simulink model "tracker_resize"  (Simulink 6.4)
settings: Solver=ode45  StartTime=0.0  StopTime=10.0  RelTol=1e-3
libraries: vipgeotforms x3, vipsnks x2, imaqlib x1
settings Model: LastModifiedBy=Raza

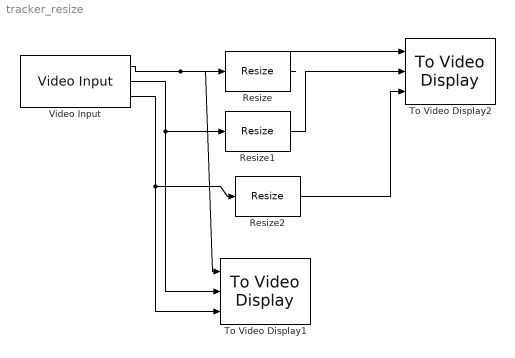
== system tracker_resize ==
  Resize : vipgeotforms/Resize  DialogController=vipDDGCreate  DialogControllerArgs=DataTag0  specify=Number of output columns and preserve aspect ratio  rfactor=[200 150]  outCols=100  outRows=25  outRowsCols=[25 35]  interp_method=Bilinear  antialias=on  prodOutputMode=Binary point scaling  prodOutputWordLength=32  prodOutputFracLength=10  roundingMode=Nearest  overflowMode=on
  Resize1 : vipgeotforms/Resize  DialogController=vipDDGCreate  DialogControllerArgs=DataTag1  specify=Number of output columns and preserve aspect ratio  rfactor=[200 150]  outCols=100  outRows=25  outRowsCols=[25 35]  interp_method=Bilinear  antialias=on  prodOutputMode=Binary point scaling  prodOutputWordLength=32  prodOutputFracLength=10  roundingMode=Nearest  overflowMode=on
  Resize2 : vipgeotforms/Resize  DialogController=vipDDGCreate  DialogControllerArgs=DataTag2  specify=Number of output columns and preserve aspect ratio  rfactor=[200 150]  outCols=100  outRows=25  outRowsCols=[25 35]  interp_method=Bilinear  antialias=on  prodOutputMode=Binary point scaling  prodOutputWordLength=32  prodOutputFracLength=10  roundingMode=Nearest  overflowMode=on
  To Video Display1 : vipsnks/To Video Display  inputType=RGB  OutputDevice=On-screen video monitor  fullScreen=off  videoWindowX=61  videoWindowY=63  saveWindowSize=off  videoWindowWidth=776  videoWindowHeight=603
  To Video Display2 : vipsnks/To Video Display  inputType=RGB  OutputDevice=On-screen video monitor  fullScreen=off  videoWindowX=44  videoWindowY=41  saveWindowSize=off  videoWindowWidth=146  videoWindowHeight=125
  Video Input : imaqlib/Video Input  DialogController=imaqcreatedialog  DialogControllerArgs=DataTag3  VideoDeviceMenu=1 (Bt878 TV Card)  VideoDevice=1 (Bt878 TV Card)  VideoStreamFormatMenu=RGB24_768x576  VideoStreamFormat=RGB555_768x576  VideoFrameSizeMenu=INPUTSIZE  VideoFrameSize=INPUTSIZE  FrameRate=5 fps  DataType=double
  wires:
  Resize/1 -> To Video Display2/1
  Resize1/1 -> To Video Display2/2
  Resize2/1 -> To Video Display2/3
  Video Input/1 -> Resize/1, To Video Display1/1
  Video Input/2 -> Resize1/1, To Video Display1/2
  Video Input/3 -> Resize2/1, To Video Display1/3
